simulink subsystem "Odometria"  (R2023b)
settings: Solver=VariableStepAuto  StartTime=0.0  StopTime=10.0  RelTol=1e-3
undefined symbols (not defined in the file): DiscIntNeverNeededParam
settings Model: Creator=Usuario  LastModifiedBy=Usuario

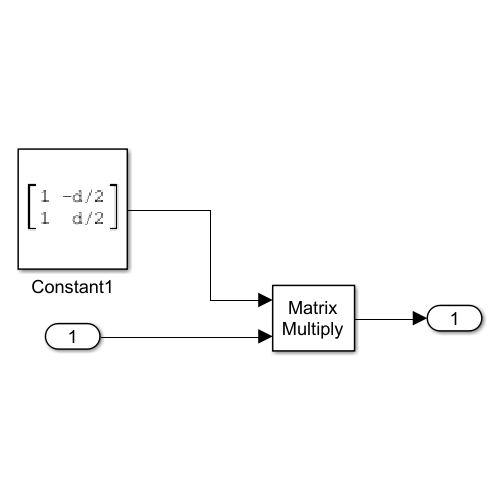
[thumbnail: Simulink's stored preview of the top-level diagram]
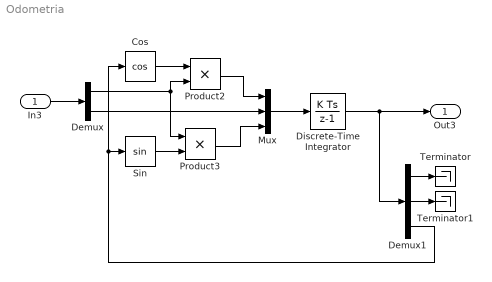
== system Odometria ==
  In3 : Inport
  Cos : Trigonometry  Operator=cos
  Demux : Demux  Outputs=2
  Demux1 : Demux  Outputs=3
  Discrete-Time Integrator : DiscreteIntegrator  SampleTime=-1  ICPrevOutput=DiscIntNeverNeededParam  ICPrevScaledInput=DiscIntNeverNeededParam
  Mux : Mux  Inputs=3
  Product2 : Product
  Product3 : Product
  Sin : Trigonometry
  Terminator : Terminator
  Terminator1 : Terminator
  Out3 : Outport
  wires:
  Demux1/1 -> Terminator/1
  Demux/2 -> Mux/2
  In3/1 -> Demux/1
  Demux1/3 -> Sin/1, Cos/1
  Demux/1 -> Product3/1, Product2/2
  Discrete-Time Integrator/1 -> Out3/1, Demux1/1
  Sin/1 -> Product3/2
  Product2/1 -> Mux/1
  Mux/1 -> Discrete-Time Integrator/1
  Cos/1 -> Product2/1
  Demux1/2 -> Terminator1/1
  Product3/1 -> Mux/3
